simulink model "JsCbM_model"  (R2023b)
settings: Solver=FixedStepAuto  StartTime=0.0  StopTime=15  FixedStep=1e-4  RelTol=1e-3
model workspace (MAT data in the model file):
  J = 5
  Ld = 0.25
  Lg = 4
  Lgq = 0.8
  Rb = 70.1
  Rd = 1.1
libraries: SignalEditorBlockLib x1
settings Model: Creator=ivanz  LastModifiedBy=ivanz

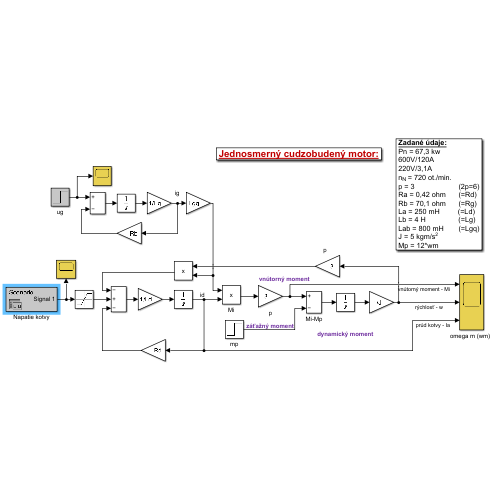
[thumbnail: Simulink's stored preview of the top-level diagram]
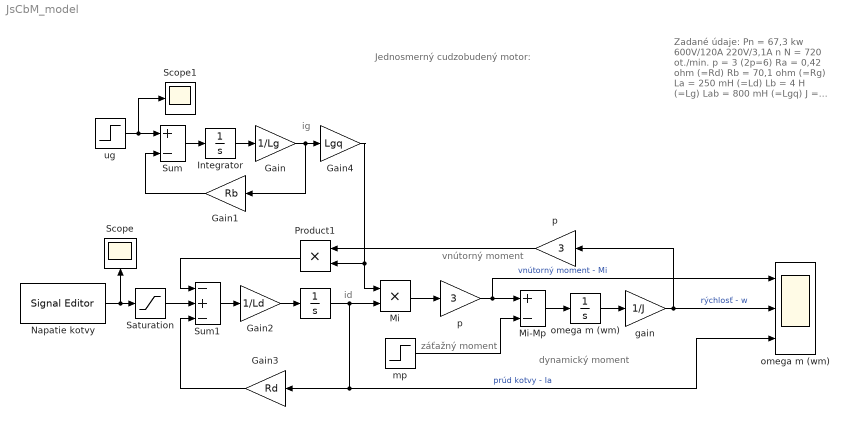
== system JsCbM_model ==
  note: vnútorný moment
  note: id
  note: ig
  note: Zadané údaje:
      | Pn = 67,3 kw
      | 600V/120A
      | 220V/3,1A
      | n N = 720 ot./min.
      | p = 3 (2p=6)
      | Ra = 0,42 ohm (=Rd)
      | Rb = 70,1 ohm (=Rg)
      | La = 250 mH (=Ld)
      | Lb = 4 H (=Lg)
      | Lab = 800 mH (=Lgq)
      | J = 5 kgm/s 2
      | Mp = 12*wm
  note: Jednosmerný cudzobudený motor:
  note: záťažný moment
  note: dynamický moment
  " " : Integrator
  " gain" : Gain  Gain=1/J
  Gain : Gain  Gain=1/Lg
  Gain1 : Gain  Gain=Rb
  Gain2 : Gain  Gain=1/Ld
  Gain3 : Gain  Gain=Rd
  Gain4 : Gain  Gain=Lgq
  Integrator : Integrator
  Mi : Product
  Mi-Mp : Sum  Inputs=+-
  Napatie kotvy : SignalEditorBlockLib/Signal Editor  FileName=C:\Users\ivanz\Desktop\DDES skúška\napatie_kotvy.mat  ActiveScenario=Scenario  ActiveSignal=Signal 1  IsBus=off  OutputBusObjectStr=Bus: BusObject  SampleTime=1e-4  ZeroCross=off  OutputAfterFinalValue=Setting to zero  Unit=inherit  PreserveSignalName=on  ApplySigPropsToAllScenarios=on  ApplySigPropsToAllSignals=on
  Product1 : Product
  Saturation : Saturate  UpperLimit=600  LowerLimit=0.5
  Scope : Scope
  Scope1 : Scope
  Sum : Sum  Inputs=+-
  Sum1 : Sum  Inputs=-+-
  mp : Step  Time=10  After=12*75  SampleTime=0
  omega m (wm) : Integrator
  "omega m (wm)  " : Scope  NumInputPorts=3
  p : Gain  Gain=3
  "p   " : Gain  Gain=3
  ug : Step  Time=0  Before=220  After=220  SampleTime=0
  wires:
  Sum/1 -> Integrator/1
  Integrator/1 -> Gain/1
  Gain1/1 -> Sum/2
  Sum1/1 -> Gain2/1
  " "/1 -> Mi/2, Gain3/1, "omega m (wm)  "/3  "prúd kotvy - Ia"
  Gain2/1 -> " "/1
  Gain3/1 -> Sum1/3
  Gain4/1 -> Product1/2, Mi/1
  Mi/1 -> p/1
  p/1 -> "omega m (wm)  "/1, Mi-Mp/1  "vnútorný moment - Mi"
  mp/1 -> Mi-Mp/2
  Mi-Mp/1 -> omega m (wm)/1
  " gain"/1 -> "p   "/1, "omega m (wm)  "/2  "rýchlosť - w"
  "p   "/1 -> Product1/1
  Product1/1 -> Sum1/1
  Saturation/1 -> Sum1/2
  Gain/1 -> Gain4/1, Gain1/1
  omega m (wm)/1 -> " gain"/1
  ug/1 -> Scope1/1, Sum/1
  Napatie kotvy/1 -> Saturation/1, Scope/1
